simulink model "DZ_AC_estFOC"  (R2019b)
settings: Solver=VariableStepAuto  StartTime=0.0  StopTime=70  RelTol=1e-3
undefined symbols (not defined in the file): alfa_beta, beta, fr_n, j, J, k_comp, ki_f, ki_I, ki_m, kp_f, kp_I, kp_m, Lkm, Lks, magnitude, n0, np, rad_to_rpm, Rr, Rs, sigbuilder_block, T_1_amp, T_amp, tau_f
libraries: simulink x2
settings Model: Creator=denni  LastModifiedBy=denniszanutto

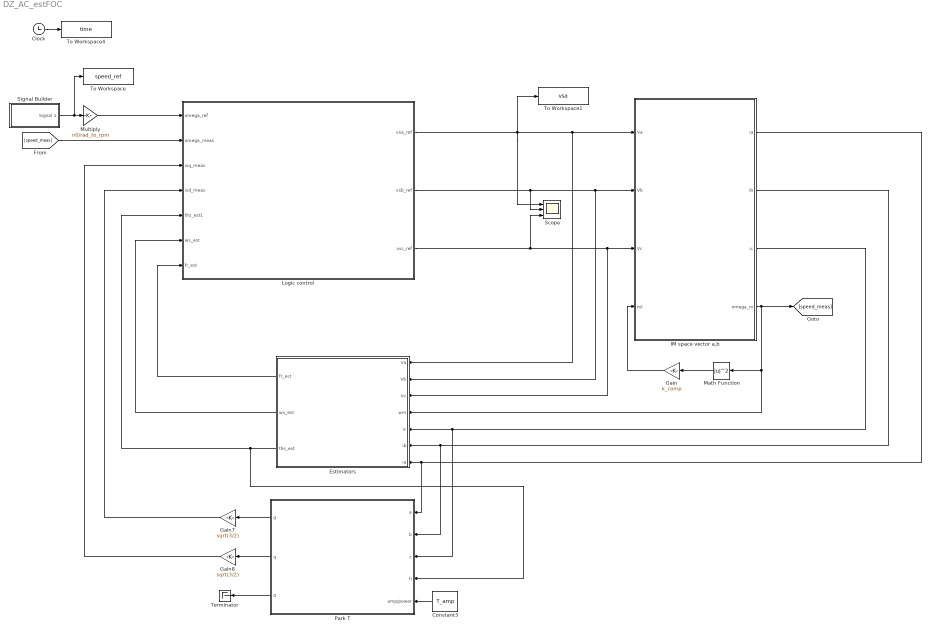
== system DZ_AC_estFOC ==
  Clock : Clock
  Constant3 : Constant  Value=T_amp
  Estimators : Subsystem
  Gain : Gain  Gain=k_comp
  Gain7 : Gain  Gain=sqrt(3/2)
  Gain8 : Gain  Gain=sqrt(3/2)
  IM space vector a,b : Subsystem
  "Logic control " : Subsystem
  Math Function : Math  Operator=magnitude^2  SignedPower=off  SaturateOnIntegerOverflow=on
  Multiply : Gain  Gain=n0/rad_to_rpm
  Park T : Subsystem
  Scope : Scope  NumInputPorts=3
  Signal Builder : Subsystem  Tag=STV Subsys  LoadFcn=sigbuilder_block('load');  StartFcn=sigbuilder_block('start');  StopFcn=sigbuilder_block('stop');  ClipboardFcn=sigbuilder_block('clipboard');  mask(Sigbuilder block){tuvar=[0:10]}
      mask help: Simulink:masks:SigbuilderBlock_MD
      mask init:
      | if ~strcmp(get_param(bdroot(gcbh),'SimulationStatus'),'stopped') tuvar = sigbuilder_block('maskInit'); end
      settings: CopyFcn=sigbuilder_block('copy');  DeleteFcn=sigbuilder_block('delete');  ModelCloseFcn=sigbuilder_block('modelClose');  PreSaveFcn=sigbuilder_block('preSave');  PauseFcn=sigbuilder_block('pause');  ContinueFcn=sigbuilder_block('continue');  NameChangeFcn=sigbuilder_block('namechange');  OpenFcn=sigbuilder_block('open',[437.6 199.2 550.4 400 ]);  CloseFcn=sigbuilder_block('close');
      mask Display: plot(0, 0, 100, 100,[2, 2, 32, 32, 2], [68, 8, 8, 68, 68],[32, 2], [38, 38], [32, 19, 2],[53, 60, 44], [32, 17, 17, 2],[16, 16, 31, 31]);txt = getActiveGroup(gcbh);text(2, 100, txt,'verticalAlignment', 'top');
  Terminator : Terminator
  To Workspace : ToWorkspace  VariableName=speed_ref  SaveFormat=Timeseries  SampleTime=-1
  To Workspace1 : ToWorkspace  VariableName=vsa  SaveFormat=Timeseries  SampleTime=-1
  To Workspace4 : ToWorkspace  VariableName=time  SaveFormat=Timeseries  SampleTime=-1
  wires:
  Gain/1 -> IM space vector a,b/4(ml)
  "Logic control "/3(vsc_ref) -> Estimators/3(Vc), IM space vector a,b/3(Vc), Scope/3
  "Logic control "/1(vsa_ref) -> Estimators/1(Va), IM space vector a,b/1(Va), Scope/1, To Workspace1/1
  "Logic control "/2("vsb_ref ") -> Estimators/2(Vb), IM space vector a,b/2(Vb), Scope/2
  IM space vector a,b/4("omega_m ") -> [speed_meas], Estimators/4("wm "), Math Function/1
  Math Function/1 -> Gain/1
  IM space vector a,b/1(ia) -> Park T/1(a), Estimators/7(ia)
  IM space vector a,b/2(ib) -> Estimators/6(ib), Park T/2(b)
  IM space vector a,b/3(ic) -> Estimators/5(ic), Park T/3("c ")
  Estimators/1("fr_est ") -> "Logic control "/7(fr_est)
  Estimators/3("ths_est ") -> Park T/4(fi), "Logic control "/5(ths_est1)
  Estimators/2("ws_est ") -> "Logic control "/6(ws_est)
  Signal Builder/1(Signal 1) -> To Workspace/1, Multiply/1
  Multiply/1 -> "Logic control "/1(omega_ref)
  Gain8/1 -> "Logic control "/3(isq_meas)
  Gain7/1 -> "Logic control "/4("isd_meas ")
  Park T/1(d) -> Gain7/1
  Park T/3(0) -> Terminator/1
  Park T/2("q ") -> Gain8/1
  Constant3/1 -> Park T/5("amp/power ")
  [speed_meas] -> "Logic control "/2(omega_meas)
  Clock/1 -> To Workspace4/1

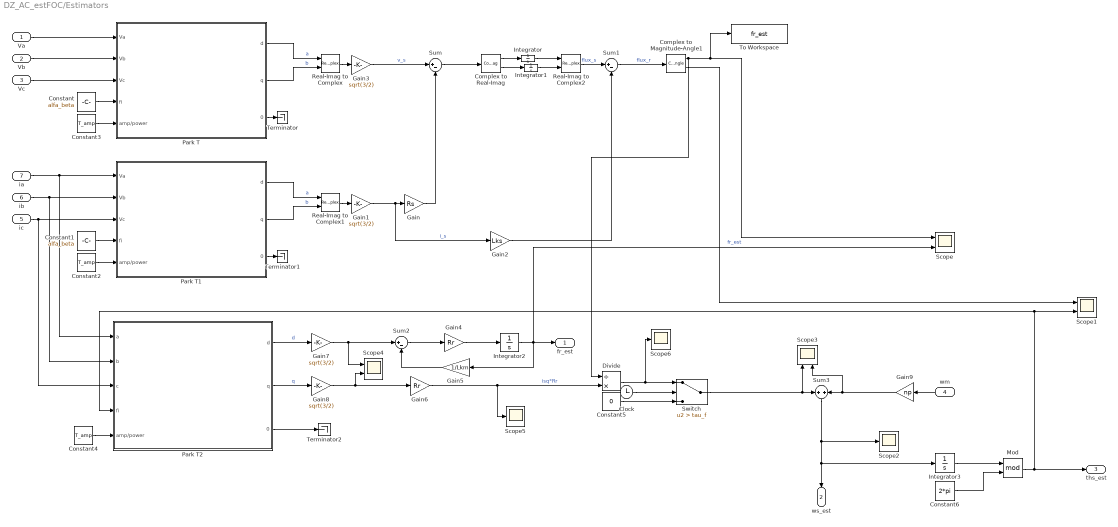
== system DZ_AC_estFOC/Estimators ==
  Va : Inport
  Vb : Inport  Port=2
  Vc : Inport  Port=3
  "wm " : Inport  Port=4
  ic : Inport  Port=5
  ib : Inport  Port=6
  ia : Inport  Port=7
  Clock : Clock
  Complex to Magnitude-Angle1 : ComplexToMagnitudeAngle
  Complex to Real-Imag : ComplexToRealImag
  Constant : Constant  Value=alfa_beta
  Constant1 : Constant  Value=alfa_beta
  Constant2 : Constant  Value=T_amp
  Constant3 : Constant  Value=T_amp
  Constant4 : Constant  Value=T_amp
  Constant5 : Constant  Value=0
  Constant6 : Constant  Value=2*pi
  Divide : Product  Inputs=/*
  Gain : Gain  Gain=Rs
  Gain{1,3,7..8} (4 alike) : Gain  Gain=sqrt(3/2)
  Gain2 : Gain  Gain=Lks
  Gain4 : Gain  Gain=Rr
  Gain5 : Gain  Gain=1/Lkm
  Gain6 : Gain  Gain=Rr
  Gain9 : Gain  Gain=np
  Integrator{,1..3} (4 alike) : Integrator
  Mod : Math  Operator=mod  SignedPower=off  SaturateOnIntegerOverflow=on
  Park T : Subsystem
  Park T1 : Subsystem
  Park T2 : Subsystem
  Real-Imag to Complex : RealImagToComplex
  Real-Imag to Complex1 : RealImagToComplex
  Real-Imag to Complex2 : RealImagToComplex
  Scope{,1,3..4} (4 alike) : Scope  NumInputPorts=2
  Scope2 : Scope
  Scope5 : Scope
  Scope6 : Scope
  Sum : Sum  Inputs=|+-
  Sum1 : Sum  Inputs=|+-
  Sum2 : Sum  Inputs=|+-
  Sum3 : Sum
  Switch : Switch  Criteria=u2 > Threshold  Threshold=tau_f
  Terminator : Terminator
  Terminator1 : Terminator
  Terminator2 : Terminator
  To Workspace : ToWorkspace  VariableName=fr_est  SaveFormat=Timeseries  SampleTime=-1
  "fr_est " : Outport
  "ws_est " : Outport  Port=2
  "ths_est " : Outport  Port=3
  wires:
  Real-Imag to Complex/1 -> Gain3/1
  Va/1 -> Park T/1(Va)
  Constant/1 -> Park T/4(fi)
  Vc/1 -> Park T/3("Vc ")
  Park T/1(d) -> Real-Imag to Complex/1  "a"
  Constant3/1 -> Park T/5("amp/power ")
  Park T/2("q ") -> Real-Imag to Complex/2  "b"
  Vb/1 -> Park T/2(Vb)
  Gain3/1 -> Sum/1  "v_s"
  Park T/3(0) -> Terminator/1
  Real-Imag to Complex1/1 -> Gain1/1
  ia/1 -> Park T1/1(Va), Park T2/1(a)
  Constant1/1 -> Park T1/4(fi)
  ic/1 -> Park T2/3("c "), Park T1/3("Vc ")
  Park T1/1(d) -> Real-Imag to Complex1/1  "a"
  Constant2/1 -> Park T1/5("amp/power ")
  Park T1/2("q ") -> Real-Imag to Complex1/2  "b"
  ib/1 -> Park T1/2(Vb), Park T2/2(b)
  Gain1/1 -> Gain2/1, Gain/1  "i_s"
  Park T1/3(0) -> Terminator1/1
  Gain/1 -> Sum/2
  Complex to Real-Imag/1 -> Integrator/1
  Sum/1 -> Complex to Real-Imag/1
  Integrator/1 -> Real-Imag to Complex2/1
  Integrator1/1 -> Real-Imag to Complex2/2
  Complex to Real-Imag/2 -> Integrator1/1
  Real-Imag to Complex2/1 -> Sum1/1  "flux_s"
  Gain2/1 -> Sum1/2
  Sum1/1 -> Complex to Magnitude-Angle1/1  "flux_r"
  Complex to Magnitude-Angle1/1 -> Divide/1, To Workspace/1, Scope/1
  Complex to Magnitude-Angle1/2 -> Scope1/1
  Gain7/1 -> Scope4/1, Sum2/1
  Park T2/1(d) -> Gain7/1  "d"
  Park T2/2("q ") -> Gain8/1  "q"
  Park T2/3(0) -> Terminator2/1
  Constant4/1 -> Park T2/5("amp/power ")
  Gain4/1 -> Integrator2/1
  Gain8/1 -> Scope4/2, Gain6/1
  Integrator2/1 -> Gain5/1, "fr_est "/1, Scope/2  "fr_est"
  Sum2/1 -> Gain4/1
  Gain5/1 -> Sum2/2
  Gain6/1 -> Scope5/1, Divide/2  "isq*Rr"
  Sum3/1 -> "ws_est "/1, Integrator3/1, Scope2/1
  "wm "/1 -> Gain9/1
  Divide/1 -> Switch/1, Scope6/1
  Switch/1 -> Scope3/1, Sum3/1
  Gain9/1 -> Scope3/2, Sum3/2
  Constant5/1 -> Switch/3
  Constant6/1 -> Mod/2
  Integrator3/1 -> Mod/1
  Mod/1 -> "ths_est "/1, Park T2/4(fi), Scope1/2
  Clock/1 -> Switch/2

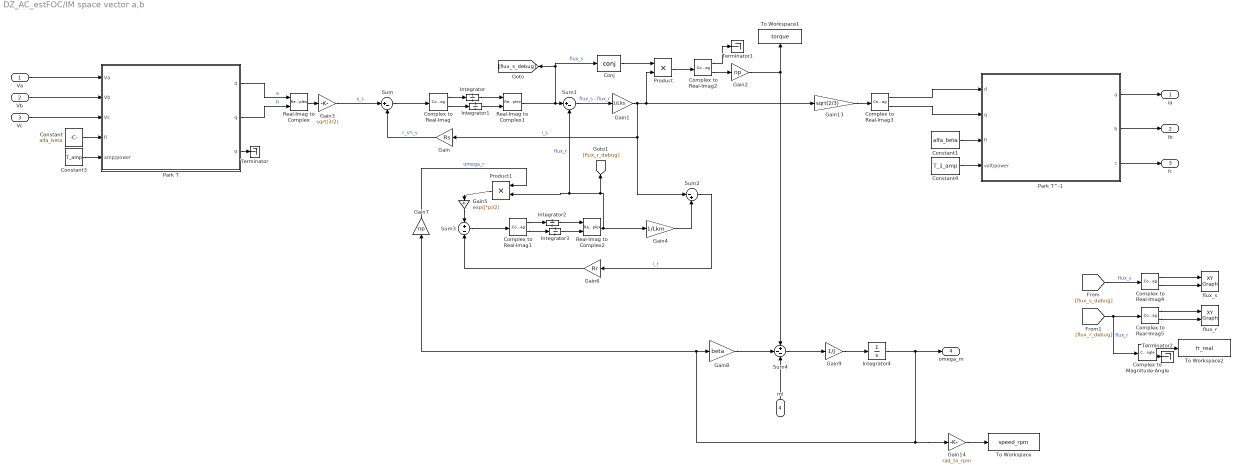
== system DZ_AC_estFOC/IM space vector a,b ==
  Va : Inport
  Vb : Inport  Port=2
  Vc : Inport  Port=3
  ml : Inport  Port=4
  Complex to Magnitude-Angle : ComplexToMagnitudeAngle
  Complex to Real-Imag{,1..5} (6 alike) : ComplexToRealImag
  Conj : Math  Operator=conj  SignedPower=off  SaturateOnIntegerOverflow=on
  Constant : Constant  Value=alfa_beta
  Constant1 : Constant  Value=alfa_beta
  Constant3 : Constant  Value=T_amp
  Constant4 : Constant  Value=T_1_amp
  Gain : Gain  Gain=Rs
  Gain1 : Gain  Gain=1/Lks
  Gain13 : Gain  Gain=sqrt(2/3)
  Gain14 : Gain  Gain=rad_to_rpm
  Gain2 : Gain  Gain=np
  Gain3 : Gain  Gain=sqrt(3/2)
  Gain4 : Gain  Gain=1/Lkm
  Gain5 : Gain  Gain=exp(j*pi/2)
  Gain6 : Gain  Gain=Rr
  Gain7 : Gain  Gain=np
  Gain8 : Gain  Gain=beta
  Gain9 : Gain  Gain=1/J
  Integrator{,1..4} (5 alike) : Integrator
  Park T : Subsystem
  Park T^-1 : Subsystem
  Product : Product
  Product1 : Product
  Real-Imag to Complex : RealImagToComplex
  Real-Imag to Complex1 : RealImagToComplex
  Real-Imag to Complex2 : RealImagToComplex
  Sum : Sum  Inputs=|+-
  Sum1 : Sum  Inputs=|+-
  Sum2 : Sum  Inputs=|-+
  Sum3 : Sum  Inputs=+-
  Sum4 : Sum  Inputs=+--
  Terminator : Terminator
  Terminator1 : Terminator
  Terminator2 : Terminator
  To Workspace : ToWorkspace  VariableName=speed_rpm  SaveFormat=Timeseries  SampleTime=-1
  To Workspace1 : ToWorkspace  VariableName=torque  SaveFormat=Timeseries  SampleTime=-1
  To Workspace2 : ToWorkspace  VariableName=fr_real  SaveFormat=Timeseries  SampleTime=-1
  flux_r : simulink/Sinks/XY Graph  xmin=-4  xmax=4  ymin=-4  ymax=4  st=-1
  flux_s : simulink/Sinks/XY Graph  xmin=-5  xmax=5  ymin=-5  ymax=5  st=-1
  ia : Outport
  ib : Outport  Port=2
  ic : Outport  Port=3
  "omega_m " : Outport  Port=4
  wires:
  Vc/1 -> Park T/3("Vc ")
  Constant/1 -> Park T/4(fi)
  Constant3/1 -> Park T/5("amp/power ")
  Park T/1(d) -> Real-Imag to Complex/1  "a"
  Park T/2("q ") -> Real-Imag to Complex/2  "b"
  Real-Imag to Complex/1 -> Gain3/1
  Sum/1 -> Complex to Real-Imag/1
  Complex to Real-Imag/1 -> Integrator/1
  Complex to Real-Imag/2 -> Integrator1/1
  Integrator/1 -> Real-Imag to Complex1/1
  Integrator1/1 -> Real-Imag to Complex1/2
  Gain/1 -> Sum/2  "r_s*i_s"
  Real-Imag to Complex1/1 -> Conj/1, [flux_s_debug], Sum1/1  "flux_s"
  Sum1/1 -> Gain1/1  "flux_s - flux_r"
  Gain1/1 -> Product/2, Gain13/1, Sum2/1, Gain/1  "i_s"
  Conj/1 -> Product/1
  Complex to Real-Imag1/1 -> Integrator2/1
  Complex to Real-Imag1/2 -> Integrator3/1
  Integrator2/1 -> Real-Imag to Complex2/1
  Integrator3/1 -> Real-Imag to Complex2/2
  Gain4/1 -> Sum2/2
  Real-Imag to Complex2/1 -> [flux_r_debug], Product1/2, Sum1/2, Gain4/1  "flux_r"
  Sum3/1 -> Complex to Real-Imag1/1
  Gain5/1 -> Sum3/1
  Product1/1 -> Gain5/1
  Gain6/1 -> Sum3/2
  Sum2/1 -> Gain6/1  "i_r"
  ml/1 -> Sum4/3
  Sum4/1 -> Gain9/1
  Gain9/1 -> Integrator4/1
  Product/1 -> Complex to Real-Imag2/1
  Integrator4/1 -> "omega_m "/1, Gain14/1, Gain7/1, Gain8/1
  Gain2/1 -> To Workspace1/1, Sum4/1
  Va/1 -> Park T/1(Va)
  Vb/1 -> Park T/2(Vb)
  Gain8/1 -> Sum4/2
  Complex to Real-Imag2/2 -> Gain2/1
  Gain3/1 -> Sum/1  "v_s"
  Gain7/1 -> Product1/1  "omega_r"
  Gain13/1 -> Complex to Real-Imag3/1
  Complex to Real-Imag3/2 -> Park T^-1/2(q)
  Complex to Real-Imag3/1 -> Park T^-1/1(d)
  Constant1/1 -> Park T^-1/3(fi)
  Constant4/1 -> Park T^-1/4(volt/power)
  Park T^-1/1("a ") -> ia/1
  Park T^-1/2("b ") -> ib/1
  Park T^-1/3(c) -> ic/1
  Park T/3(0) -> Terminator/1
  Complex to Real-Imag2/1 -> Terminator1/1
  [flux_s_debug] -> Complex to Real-Imag4/1  "flux_s"
  [flux_r_debug] -> Complex to Real-Imag5/1, Complex to Magnitude-Angle/1  "flux_r"
  Complex to Real-Imag4/1 -> flux_s/1
  Complex to Real-Imag4/2 -> flux_s/2
  Complex to Real-Imag5/1 -> flux_r/1
  Complex to Real-Imag5/2 -> flux_r/2
  Gain14/1 -> To Workspace/1
  Complex to Magnitude-Angle/1 -> To Workspace2/1
  Complex to Magnitude-Angle/2 -> Terminator2/1

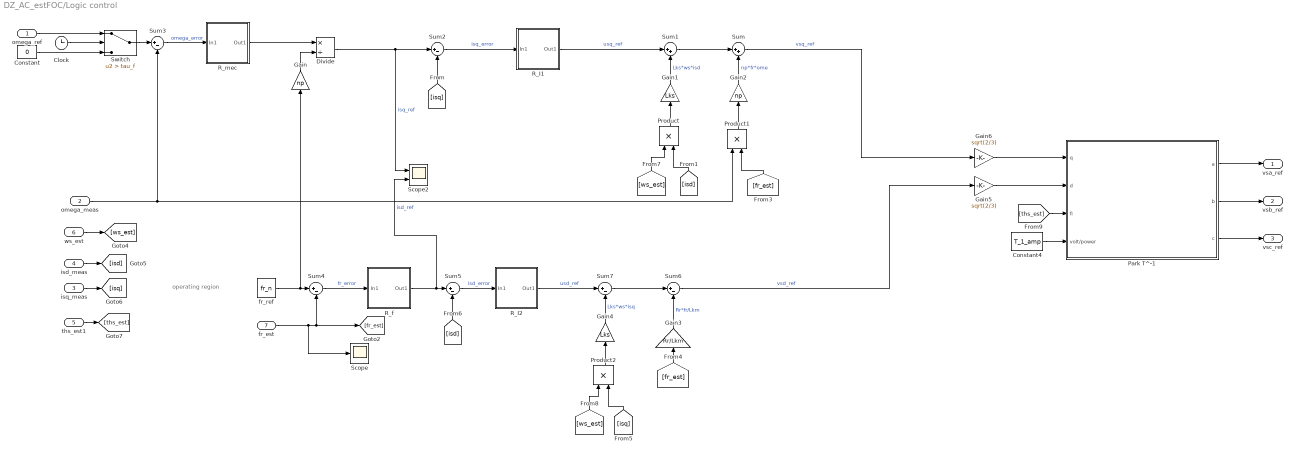
== system DZ_AC_estFOC/Logic control  ==
  note: operating region
  omega_ref : Inport
  omega_meas : Inport  Port=2
  isq_meas : Inport  Port=3
  "isd_meas " : Inport  Port=4
  ths_est1 : Inport  Port=5
  ws_est : Inport  Port=6
  fr_est : Inport  Port=7
  Clock : Clock
  Constant : Constant  Value=0
  Constant4 : Constant  Value=T_1_amp
  Divide : Product  Inputs=*/
  Gain : Gain  Gain=np
  Gain1 : Gain  Gain=Lks
  Gain2 : Gain  Gain=np
  Gain3 : Gain  Gain=Rr/Lkm
  Gain4 : Gain  Gain=Lks
  Gain5 : Gain  Gain=sqrt(2/3)
  Gain6 : Gain  Gain=sqrt(2/3)
  Park T^-1 : Subsystem
  Product : Product
  Product1 : Product
  Product2 : Product
  R_I1 : Subsystem
  R_I2 : Subsystem
  "R_f " : Subsystem
  R_mec : Subsystem
  Scope : Scope
  Scope2 : Scope  NumInputPorts=2
  Sum : Sum  Inputs=|++
  Sum1 : Sum  Inputs=|++
  Sum{2..7} (6 alike) : Sum  Inputs=|+-
  Switch : Switch  Criteria=u2 > Threshold  Threshold=tau_f
  "fr_ref " : Constant  Value=fr_n
  vsa_ref : Outport
  "vsb_ref " : Outport  Port=2
  vsc_ref : Outport  Port=3
  wires:
  Constant4/1 -> Park T^-1/4(volt/power)
  [ths_est] -> Park T^-1/3(fi)
  Sum/1 -> Gain6/1  "vsq_ref"
  Park T^-1/3(c) -> vsc_ref/1
  Sum1/1 -> Sum/1
  Sum3/1 -> R_mec/1(In1)  "omega_error"
  Gain/1 -> Divide/2
  [isq] -> Sum2/2
  Product/1 -> Gain1/1
  [isd] -> Product/2
  omega_meas/1 -> Product1/1, Sum3/2
  Product1/1 -> Gain2/1
  "fr_ref "/1 -> Gain/1, Sum4/1
  fr_est/1 -> Scope/1, [fr_est], Sum4/2
  [fr_est] -> Product1/2
  Sum4/1 -> "R_f "/1(In1)  "fr_error"
  "R_f "/1(Out1) -> Scope2/2, Sum5/1  "isd_ref"
  Sum5/1 -> R_I2/1(In1)  "isd_error"
  Sum7/1 -> Sum6/1
  R_I2/1(Out1) -> Sum7/1  "usd_ref"
  Sum6/1 -> Gain5/1  "vsd_ref"
  [fr_est] -> Gain3/1
  Park T^-1/1("a ") -> vsa_ref/1
  Park T^-1/2("b ") -> "vsb_ref "/1
  [isq] -> Product2/2
  Product2/1 -> Gain4/1
  [isd] -> Sum5/2
  ws_est/1 -> [ws_est]
  [ws_est] -> Product/1
  [ws_est] -> Product2/1
  R_I1/1(Out1) -> Sum1/1  "usq_ref"
  Sum2/1 -> R_I1/1(In1)  "isq_error"
  R_mec/1(Out1) -> Divide/1
  Gain1/1 -> Sum1/2  "Lks*ws*isd"
  Gain2/1 -> Sum/2  "np*fr*ome"
  Gain4/1 -> Sum7/2  "Lks*ws*isq"
  Gain3/1 -> Sum6/2  "Rr*fr/Lkm"
  Divide/1 -> Scope2/1, Sum2/1  "isq_ref"
  Gain6/1 -> Park T^-1/1(q)
  Gain5/1 -> Park T^-1/2(d)
  ths_est1/1 -> [ths_est]
  "isd_meas "/1 -> [isd]
  isq_meas/1 -> [isq]
  Constant/1 -> Switch/3
  omega_ref/1 -> Switch/1
  Switch/1 -> Sum3/1
  Clock/1 -> Switch/2

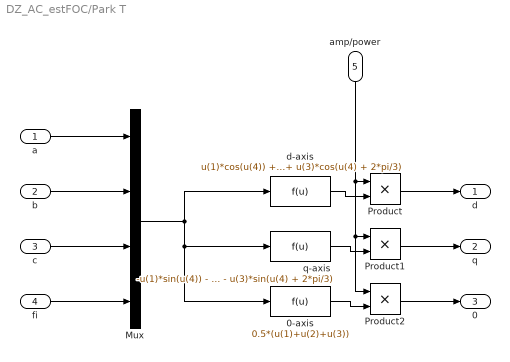
== system DZ_AC_estFOC/Park T ==
  a : Inport
  b : Inport  Port=2
  "c " : Inport  Port=3
  fi : Inport  Port=4
  "amp/power " : Inport  Port=5
  0-axis : Fcn  Expr=0.5*(u(1)+u(2)+u(3))
  Mux : Mux
  Product : Product
  Product1 : Product
  Product2 : Product
  "d-axis " : Fcn  Expr=u(1)*cos(u(4)) + u(2)*cos(u(4) -2*pi/3) + u(3)*cos(u(4) + 2*pi/3)
  q-axis : Fcn  Expr=-u(1)*sin(u(4)) - u(2)*sin(u(4) -2*pi/3) - u(3)*sin(u(4) + 2*pi/3)
  d : Outport
  "q " : Outport  Port=2
  0 : Outport  Port=3
  wires:
  fi/1 -> Mux/4
  a/1 -> Mux/1
  b/1 -> Mux/2
  "c "/1 -> Mux/3
  Mux/1 -> "d-axis "/1, q-axis/1, 0-axis/1
  Product/1 -> d/1
  "d-axis "/1 -> Product/2
  Product1/1 -> "q "/1
  q-axis/1 -> Product1/2
  0-axis/1 -> Product2/2
  Product2/1 -> 0/1
  "amp/power "/1 -> Product2/1, Product1/1, Product/1

== system DZ_AC_estFOC/Signal Builder ==
  Demux : Demux  Tag=STV Demux  Outputs=1
  FromWs : FromWorkspace  Tag=STV FromWs  VariableName=tuvar  SampleTime=0
      SigBuilderData=|
      | common.afterFinalStr = 'Extrapolate'
      | common.sampleTime = 0
      | dataSet.timeRange = [0 70]
      | dataSet.name = 'Group 1'
      | sbobj.Groups.Name = 'Group 1'
      | sbobj.Groups.Signals.Name = 'Signal 1'
      | sbobj.Groups.Signals.XData = [0 20 30 40 70]
      | sbobj.Groups.Signals.YData = [0 0.1 0.1 0.2 0.2]
      | sbobj.Groups.TimeRange = [0 70]
  Signal 1 : Outport  Tag=STV Outport
  wires:
  Demux/1 -> Signal 1/1
  FromWs/1 -> Demux/1

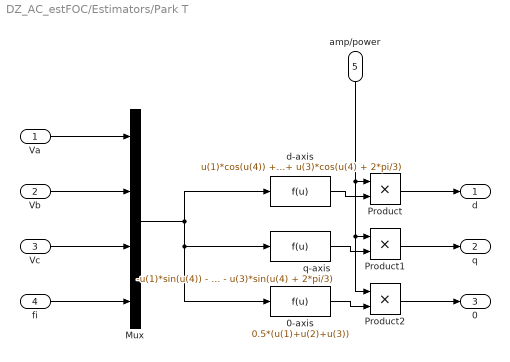
== system DZ_AC_estFOC/Estimators/Park T ==
  Va : Inport
  Vb : Inport  Port=2
  "Vc " : Inport  Port=3
  fi : Inport  Port=4
  "amp/power " : Inport  Port=5
  0-axis : Fcn  Expr=0.5*(u(1)+u(2)+u(3))
  Mux : Mux
  Product : Product
  Product1 : Product
  Product2 : Product
  "d-axis " : Fcn  Expr=u(1)*cos(u(4)) + u(2)*cos(u(4) -2*pi/3) + u(3)*cos(u(4) + 2*pi/3)
  q-axis : Fcn  Expr=-u(1)*sin(u(4)) - u(2)*sin(u(4) -2*pi/3) - u(3)*sin(u(4) + 2*pi/3)
  d : Outport
  "q " : Outport  Port=2
  0 : Outport  Port=3
  wires:
  fi/1 -> Mux/4
  Va/1 -> Mux/1
  Vb/1 -> Mux/2
  "Vc "/1 -> Mux/3
  Mux/1 -> "d-axis "/1, q-axis/1, 0-axis/1
  Product/1 -> d/1
  "d-axis "/1 -> Product/2
  Product1/1 -> "q "/1
  q-axis/1 -> Product1/2
  0-axis/1 -> Product2/2
  Product2/1 -> 0/1
  "amp/power "/1 -> Product2/1, Product1/1, Product/1

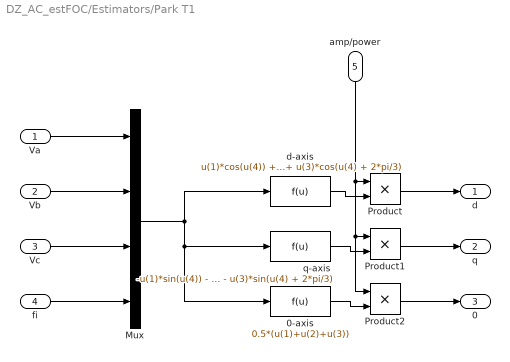
== system DZ_AC_estFOC/Estimators/Park T1 ==
  Va : Inport
  Vb : Inport  Port=2
  "Vc " : Inport  Port=3
  fi : Inport  Port=4
  "amp/power " : Inport  Port=5
  0-axis : Fcn  Expr=0.5*(u(1)+u(2)+u(3))
  Mux : Mux
  Product : Product
  Product1 : Product
  Product2 : Product
  "d-axis " : Fcn  Expr=u(1)*cos(u(4)) + u(2)*cos(u(4) -2*pi/3) + u(3)*cos(u(4) + 2*pi/3)
  q-axis : Fcn  Expr=-u(1)*sin(u(4)) - u(2)*sin(u(4) -2*pi/3) - u(3)*sin(u(4) + 2*pi/3)
  d : Outport
  "q " : Outport  Port=2
  0 : Outport  Port=3
  wires:
  fi/1 -> Mux/4
  Va/1 -> Mux/1
  Vb/1 -> Mux/2
  "Vc "/1 -> Mux/3
  Mux/1 -> "d-axis "/1, q-axis/1, 0-axis/1
  Product/1 -> d/1
  "d-axis "/1 -> Product/2
  Product1/1 -> "q "/1
  q-axis/1 -> Product1/2
  0-axis/1 -> Product2/2
  Product2/1 -> 0/1
  "amp/power "/1 -> Product2/1, Product1/1, Product/1

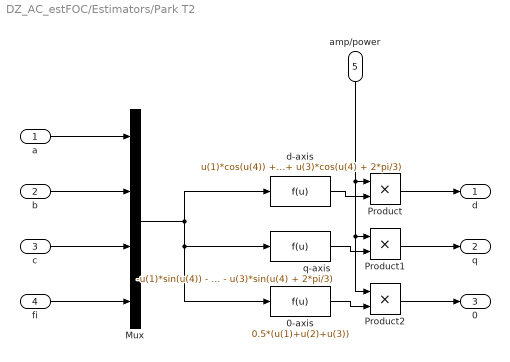
== system DZ_AC_estFOC/Estimators/Park T2 ==
  a : Inport
  b : Inport  Port=2
  "c " : Inport  Port=3
  fi : Inport  Port=4
  "amp/power " : Inport  Port=5
  0-axis : Fcn  Expr=0.5*(u(1)+u(2)+u(3))
  Mux : Mux
  Product : Product
  Product1 : Product
  Product2 : Product
  "d-axis " : Fcn  Expr=u(1)*cos(u(4)) + u(2)*cos(u(4) -2*pi/3) + u(3)*cos(u(4) + 2*pi/3)
  q-axis : Fcn  Expr=-u(1)*sin(u(4)) - u(2)*sin(u(4) -2*pi/3) - u(3)*sin(u(4) + 2*pi/3)
  d : Outport
  "q " : Outport  Port=2
  0 : Outport  Port=3
  wires:
  fi/1 -> Mux/4
  a/1 -> Mux/1
  b/1 -> Mux/2
  "c "/1 -> Mux/3
  Mux/1 -> "d-axis "/1, q-axis/1, 0-axis/1
  Product/1 -> d/1
  "d-axis "/1 -> Product/2
  Product1/1 -> "q "/1
  q-axis/1 -> Product1/2
  0-axis/1 -> Product2/2
  Product2/1 -> 0/1
  "amp/power "/1 -> Product2/1, Product1/1, Product/1

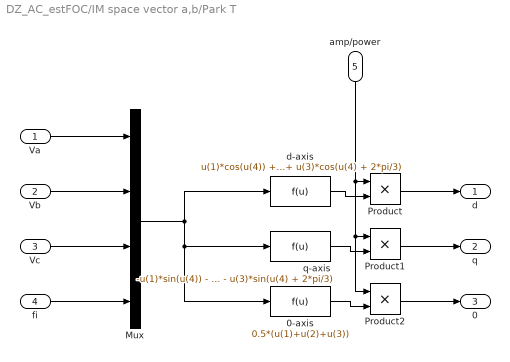
== system DZ_AC_estFOC/IM space vector a,b/Park T ==
  Va : Inport
  Vb : Inport  Port=2
  "Vc " : Inport  Port=3
  fi : Inport  Port=4
  "amp/power " : Inport  Port=5
  0-axis : Fcn  Expr=0.5*(u(1)+u(2)+u(3))
  Mux : Mux
  Product : Product
  Product1 : Product
  Product2 : Product
  "d-axis " : Fcn  Expr=u(1)*cos(u(4)) + u(2)*cos(u(4) -2*pi/3) + u(3)*cos(u(4) + 2*pi/3)
  q-axis : Fcn  Expr=-u(1)*sin(u(4)) - u(2)*sin(u(4) -2*pi/3) - u(3)*sin(u(4) + 2*pi/3)
  d : Outport
  "q " : Outport  Port=2
  0 : Outport  Port=3
  wires:
  fi/1 -> Mux/4
  Va/1 -> Mux/1
  Vb/1 -> Mux/2
  "Vc "/1 -> Mux/3
  Mux/1 -> "d-axis "/1, q-axis/1, 0-axis/1
  Product/1 -> d/1
  "d-axis "/1 -> Product/2
  Product1/1 -> "q "/1
  q-axis/1 -> Product1/2
  0-axis/1 -> Product2/2
  Product2/1 -> 0/1
  "amp/power "/1 -> Product2/1, Product1/1, Product/1

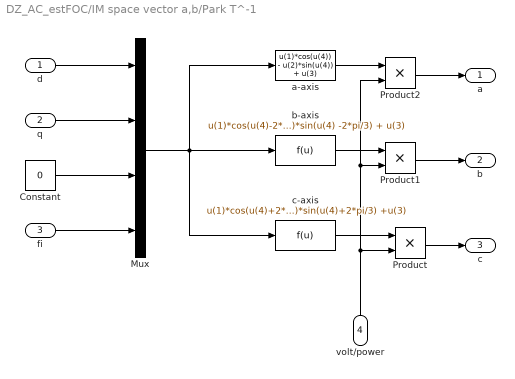
== system DZ_AC_estFOC/IM space vector a,b/Park T^-1 ==
  d : Inport
  q : Inport  Port=2
  fi : Inport  Port=3
  volt/power : Inport  Port=4
  Constant : Constant  Value=0
  Mux : Mux
  Product : Product
  Product1 : Product
  Product2 : Product
  "a-axis " : Fcn  Expr=u(1)*cos(u(4)) - u(2)*sin(u(4)) + u(3)
  b-axis : Fcn  Expr=u(1)*cos(u(4)-2*pi/3) - u(2)*sin(u(4) -2*pi/3) + u(3)
  c-axis : Fcn  Expr=u(1)*cos(u(4)+2*pi/3) -u(2)*sin(u(4)+2*pi/3) +u(3)
  "a " : Outport
  "b " : Outport  Port=2
  c : Outport  Port=3
  wires:
  fi/1 -> Mux/4
  d/1 -> Mux/1
  q/1 -> Mux/2
  Mux/1 -> c-axis/1, b-axis/1, "a-axis "/1
  Constant/1 -> Mux/3
  volt/power/1 -> Product2/2, Product1/2, Product/2
  c-axis/1 -> Product/1
  Product/1 -> c/1
  Product1/1 -> "b "/1
  b-axis/1 -> Product1/1
  Product2/1 -> "a "/1
  "a-axis "/1 -> Product2/1

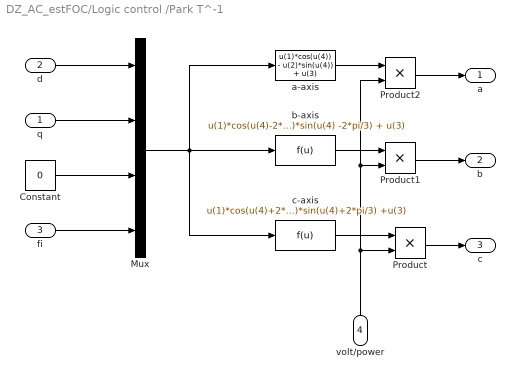
== system DZ_AC_estFOC/Logic control /Park T^-1 ==
  q : Inport
  d : Inport  Port=2
  fi : Inport  Port=3
  volt/power : Inport  Port=4
  Constant : Constant  Value=0
  Mux : Mux
  Product : Product
  Product1 : Product
  Product2 : Product
  "a-axis " : Fcn  Expr=u(1)*cos(u(4)) - u(2)*sin(u(4)) + u(3)
  b-axis : Fcn  Expr=u(1)*cos(u(4)-2*pi/3) - u(2)*sin(u(4) -2*pi/3) + u(3)
  c-axis : Fcn  Expr=u(1)*cos(u(4)+2*pi/3) -u(2)*sin(u(4)+2*pi/3) +u(3)
  "a " : Outport
  "b " : Outport  Port=2
  c : Outport  Port=3
  wires:
  fi/1 -> Mux/4
  d/1 -> Mux/1
  q/1 -> Mux/2
  Mux/1 -> c-axis/1, b-axis/1, "a-axis "/1
  Constant/1 -> Mux/3
  volt/power/1 -> Product2/2, Product1/2, Product/2
  c-axis/1 -> Product/1
  Product/1 -> c/1
  Product1/1 -> "b "/1
  b-axis/1 -> Product1/1
  Product2/1 -> "a "/1
  "a-axis "/1 -> Product2/1

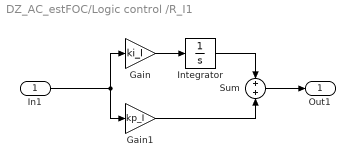
== system DZ_AC_estFOC/Logic control /R_I1 ==
  In1 : Inport
  Gain : Gain  Gain=ki_I
  Gain1 : Gain  Gain=kp_I
  Integrator : Integrator
  Sum : Sum
  Out1 : Outport
  wires:
  Gain/1 -> Integrator/1
  In1/1 -> Gain/1, Gain1/1
  Integrator/1 -> Sum/1
  Gain1/1 -> Sum/2
  Sum/1 -> Out1/1

== system DZ_AC_estFOC/Logic control /R_I2 ==
  In1 : Inport
  Gain : Gain  Gain=ki_I
  Gain1 : Gain  Gain=kp_I
  Integrator : Integrator
  Sum : Sum
  Out1 : Outport
  wires:
  Gain/1 -> Integrator/1
  In1/1 -> Gain/1, Gain1/1
  Integrator/1 -> Sum/1
  Gain1/1 -> Sum/2
  Sum/1 -> Out1/1

== system DZ_AC_estFOC/Logic control /R_f  ==
  In1 : Inport
  Gain : Gain  Gain=ki_f
  Gain1 : Gain  Gain=kp_f
  Integrator : Integrator
  Sum : Sum
  Out1 : Outport
  wires:
  In1/1 -> Gain/1, Gain1/1
  Sum/1 -> Out1/1
  Gain/1 -> Integrator/1
  Integrator/1 -> Sum/1
  Gain1/1 -> Sum/2

== system DZ_AC_estFOC/Logic control /R_mec ==
  In1 : Inport
  Gain : Gain  Gain=ki_m
  Gain1 : Gain  Gain=kp_m
  Integrator : Integrator
  Sum : Sum
  Out1 : Outport
  wires:
  In1/1 -> Gain/1, Gain1/1
  Sum/1 -> Out1/1
  Gain/1 -> Integrator/1
  Integrator/1 -> Sum/1
  Gain1/1 -> Sum/2
